simulink model "Encoder"  (R2023a)
settings: Solver=VariableStepAuto  StartTime=0.0  StopTime=10.0  RelTol=1e-3
settings Model: Creator=Artem Sannikov  LastModifiedBy=Artem Sannikov

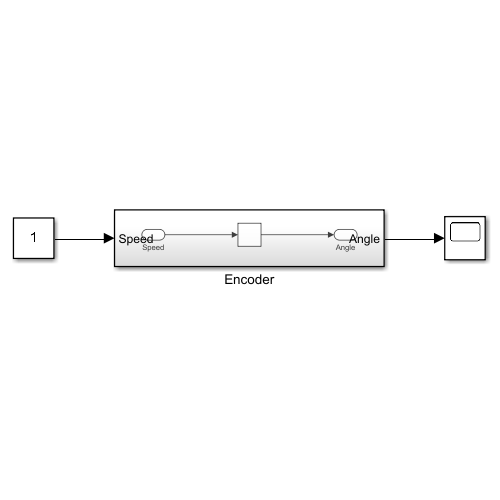
[thumbnail: Simulink's stored preview of the top-level diagram]
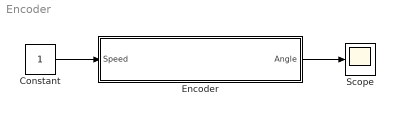
== system Encoder ==
  Constant : Constant
  Encoder : Subsystem
  Scope : Scope
  wires:
  Constant/1 -> Encoder/1(Speed)
  Encoder/1(Angle) -> Scope/1

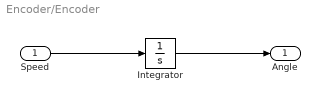
== system Encoder/Encoder ==
  Speed : Inport
  Integrator : Integrator
  Angle : Outport
  wires:
  Speed/1 -> Integrator/1
  Integrator/1 -> Angle/1
